simulink model "simscape_servo_model"  (R2020b)
settings: Solver=VariableStepAuto  StartTime=0.0  StopTime=10.0  RelTol=1e-3
libraries: fl_lib x7, nesl_utility x6, ee_lib x1
settings Model: Creator=akern  LastModifiedBy=akern

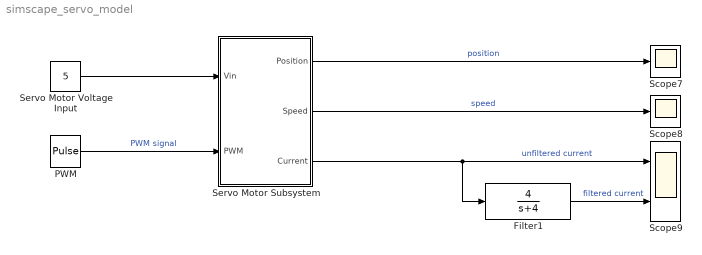
== system simscape_servo_model ==
  Filter1 : TransferFcn  Numerator=[4]  Denominator=[1 4]
  PWM : DiscretePulseGenerator  PulseType=Time based  Amplitude=5  Period=1/500  PulseWidth=50
  Scope7 : Scope
  Scope8 : Scope
  Scope9 : Scope  NumInputPorts=2
  Servo Motor Subsystem : Subsystem
  Servo Motor Voltage Input : Constant  Value=5
  wires:
  Servo Motor Subsystem/2(Speed) -> Scope8/1  "speed"
  Servo Motor Subsystem/3(Current) -> Scope9/1, Filter1/1  "unfiltered current"
  Servo Motor Voltage Input/1 -> Servo Motor Subsystem/1(Vin)
  Servo Motor Subsystem/1(Position) -> Scope7/1  "position"
  Filter1/1 -> Scope9/2  "filtered current"
  PWM/1 -> Servo Motor Subsystem/2(PWM)  "PWM signal"

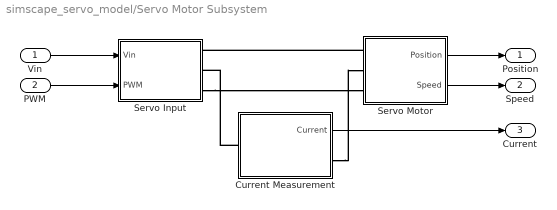
== system simscape_servo_model/Servo Motor Subsystem ==
  Vin : Inport
  PWM : Inport  Port=2
  Current Measurement : Subsystem
  Servo Input : Subsystem
  Servo Motor : Subsystem
  Position : Outport
  Speed : Outport  Port=2
  Current : Outport  Port=3
  wires:
  Servo Motor/1(Position) -> Position/1
  Vin/1 -> Servo Input/1(Vin)
  Servo Motor/2(Speed) -> Speed/1
  PWM/1 -> Servo Input/2(PWM)
  Current Measurement/1(Current) -> Current/1
  connections:
  Servo Motor/LConn1 -- Servo Input/RConn1
  Servo Input/RConn3 -- Servo Motor/LConn3
  Current Measurement/LConn1 -- Servo Input/RConn2
  Current Measurement/RConn1 -- Servo Motor/LConn2

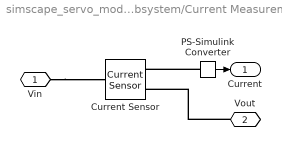
== system simscape_servo_model/Servo Motor Subsystem/Current Measurement ==
  Current Sensor : fl_lib/Electrical/Electrical Sensors/Current Sensor
  PS-Simulink Converter : nesl_utility/PS-Simulink Converter  PhysicalDomain=network_engine_domain  SubClassName=ps_output  LeftPortType=input  RightPortType=output  PseudoPeriodic=off  Frequencies=[]  Unit=inherit  AffineConversion=off
  Vin : PMIOPort  Side=Left
  Vout : PMIOPort  Port=2  Side=Right
  Current : Outport
  wires:
  PS-Simulink Converter/1 -> Current/1
  connections:
  PS-Simulink Converter/LConn1 -- Current Sensor/RConn1
  Vout/RConn1 -- Current Sensor/RConn2
  Vin/RConn1 -- Current Sensor/LConn1

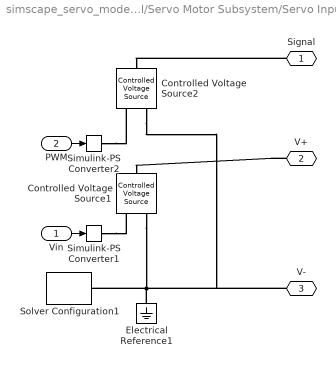
== system simscape_servo_model/Servo Motor Subsystem/Servo Input ==
  Vin : Inport
  PWM : Inport  Port=2
  Controlled Voltage Source1 : fl_lib/Electrical/Electrical Sources/Controlled Voltage Source
  Controlled Voltage Source2 : fl_lib/Electrical/Electrical Sources/Controlled Voltage Source
  Electrical Reference1 : fl_lib/Electrical/Electrical Elements/Electrical Reference
  Simulink-PS Converter1 : nesl_utility/Simulink-PS Converter  PhysicalDomain=network_engine_domain  SubClassName=ps_input  LeftPortType=input  RightPortType=output  PseudoPeriodic=off  Frequencies=[]  NoiseDistribution=none  NoiseParameters=[]  Unit=1  AffineConversion=off  FilteringAndDerivatives=provide  SimscapeFilterOrder=1  InputFilterTimeConstant=0.001  UdotUserProvided=0
  Simulink-PS Converter2 : nesl_utility/Simulink-PS Converter  PhysicalDomain=network_engine_domain  SubClassName=ps_input  LeftPortType=input  RightPortType=output  PseudoPeriodic=off  Frequencies=[]  NoiseDistribution=none  NoiseParameters=[]  Unit=1  AffineConversion=off  FilteringAndDerivatives=provide  SimscapeFilterOrder=1  InputFilterTimeConstant=0.001  UdotUserProvided=0
  Solver Configuration1 : nesl_utility/Solver Configuration  PhysicalDomain=network_engine_domain  SubClassName=solver  LeftPortType=input  RightPortType=generic  Tones=[]  Harmonics=[]  SimulateNoise=off  Profile=off  UseLocalSampling=off  EnableSwitchedLinearOptims=on  FrequencyDomain=off  UseCCode=off  RelTol=0.001  AbsTol=1e-06  MinStep=1e-09  ToWorkspace=off  RevertToSquareIcSolve=off  NumHomotopyIterations=100  PhasorMode=off  PhasorModeNumHarmonics=1  DoDC=off  ResidualTolerance=1e-09  UseLocalSolver=off  LocalSolverChoice=NE_BACKWARD_EULER_ADVANCER  LocalSolverSampleTime=0.001  DoFixedCost=off  MaxNonlinIter=3  MaxModeIter=2  ComputeImpulses=off  ImpulseIterations=2  LinearAlgebra=auto  EquationFormulation=NE_TIME_EF  DelaysMemoryBudget=1024  AutomaticFiltering=on  FilteringTimeConstant=0.001  PartitionStorageMethod=AS_NEEDED  PartitionMemoryBudget=1024  PartitionMethod=ROBUST
  Signal : PMIOPort  Side=Right
  V+ : PMIOPort  Port=2  Side=Right
  V- : PMIOPort  Port=3  Side=Right
  wires:
  PWM/1 -> Simulink-PS Converter2/1
  Vin/1 -> Simulink-PS Converter1/1
  connections:
  Controlled Voltage Source1/RConn2 -- Electrical Reference1/LConn1 -- Solver Configuration1/RConn1 -- Controlled Voltage Source2/RConn2 -- V-/RConn1
  Simulink-PS Converter1/RConn1 -- Controlled Voltage Source1/RConn1
  Signal/RConn1 -- Controlled Voltage Source2/LConn1
  Simulink-PS Converter2/RConn1 -- Controlled Voltage Source2/RConn1
  V+/RConn1 -- Controlled Voltage Source1/LConn1

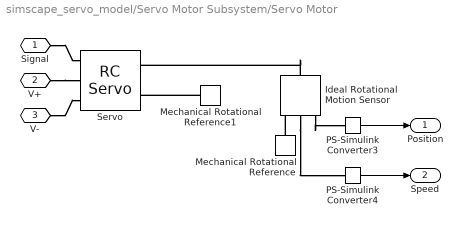
== system simscape_servo_model/Servo Motor Subsystem/Servo Motor ==
  Ideal Rotational Motion Sensor : fl_lib/Mechanical/Mechanical Sensors/Ideal Rotational Motion Sensor  wrap_angle=simscape.enum.onoff.off  offset=0 rad
  Mechanical Rotational Reference : fl_lib/Mechanical/Rotational Elements/Mechanical Rotational Reference
  Mechanical Rotational Reference1 : fl_lib/Mechanical/Rotational Elements/Mechanical Rotational Reference
  PS-Simulink Converter3 : nesl_utility/PS-Simulink Converter  PhysicalDomain=network_engine_domain  SubClassName=ps_output  LeftPortType=input  RightPortType=output  PseudoPeriodic=off  Frequencies=[]  Unit=inherit  AffineConversion=off
  PS-Simulink Converter4 : nesl_utility/PS-Simulink Converter  PhysicalDomain=network_engine_domain  SubClassName=ps_output  LeftPortType=input  RightPortType=output  PseudoPeriodic=off  Frequencies=[]  Unit=inherit  AffineConversion=off
  Servo : ee_lib/Electromechanical/Brushed Motors/RC Servo  stall_torque=2.4 kg*cm  time_60=0.28 s  nominal_voltage=4.8 V  rotational_range=[0, 180] deg  pulse_width_range=[550, 2330] us  threshold=3 V  R_s=18 kOhm  resolution=0.1 deg  angle_meas_error=0 deg  backdrive_torque=0.5 kg*cm  ratio=320  inertia=0.01 g*cm^2  endstop_angles=[-5, 185] deg  endstop_stiffness=1e6 N*m/rad  endstop_damping=0.01 N*m/(rad/s)  enable_faults=0  fault_action=1  fault_type=1  enable_temporal_fault=0  t_fault=1 s  enable_behavioral_fault=0  max_permissible_current=1 A  t_fail_on_current=1 s  angle_specify=off  angle_priority=High  angle=90 deg  angle_nominal_specify=off  angle_nominal_unit=deg  angle_nominal_value=1  w_specify=off  w_priority=High  w=0 deg/s  w_nominal_specify=off  w_nominal_unit=deg/s  w_nominal_value=1  torque_specify=off  torque_priority=None  torque=0 N*m  torque_nominal_specify=off  torque_nominal_unit=N*m  torque_nominal_value=1  pulse_width_specify=off  pulse_width_priority=Low  pulse_width=1.5 ms  i_specify=off  i_priority=None  i=0 A  i_nominal_specify=off  i_nominal_unit=A  i_nominal_value=1  i_s_specify=off  i_s_priority=None  i_s=0 A  i_s_nominal_specify=off  i_s_nominal_unit=A  i_s_nominal_value=1  motor_torque_specify=off  motor_torque_priority=None  motor_torque=0 N*m  motor_torque_nominal_specify=off  motor_torque_nominal_unit=N*m  motor_torque_nominal_value=1  power_dissipated_specify=off  power_dissipated_priority=None  power_dissipated=0 W  power_dissipated_nominal_specify=off  power_dissipated_nominal_unit=W  power_dissipated_nominal_value=1  angle_demand_specify=off  angle_demand_priority=None  angle_demand=90 deg  angle_demand_nominal_specify=off  angle_demand_nominal_unit=deg  angle_demand_nominal_value=1  faulted_specify=off  faulted_priority=None  faulted=0  faulted_nominal_specify=off  faulted_nominal_unit=1  faulted_nominal_value=1
      settings: SourceProductBaseCode=PS  InternalSimscapePortConfiguration="{\"Bottom\":[],\"Left\":[{\"id\":\"s\",\"label\":\"s\",\"type\":\"foundation.electrical.electrical\"},{\"id\":\"p\",\"label\":\"+\",\"type\":\"foundation.electrical.electrical\"},{\"id\":\"n\",\"label\":\"-\",\"type\":\"foundation.electrical.electrical\"}],\"Right\":[{\"id\":\"R\",\"label\":\"R\",\"type\":\"foundation.mechanical.rotational.rotational\"},{\"id\":\"C\",\"label\":\"C\",\"type\":\"foundation.mechanical.rotational.rotational\"}],\"Top\":[]}"
  Signal : PMIOPort  Side=Left
  V+ : PMIOPort  Port=2  Side=Left
  V- : PMIOPort  Port=3  Side=Left
  Position : Outport
  Speed : Outport  Port=2
  wires:
  PS-Simulink Converter3/1 -> Position/1
  PS-Simulink Converter4/1 -> Speed/1
  connections:
  Signal/RConn1 -- Servo/LConn1
  V-/RConn1 -- Servo/LConn3
  Ideal Rotational Motion Sensor/RConn2 -- PS-Simulink Converter4/LConn1
  Mechanical Rotational Reference/LConn1 -- Ideal Rotational Motion Sensor/RConn1
  Ideal Rotational Motion Sensor/RConn3 -- PS-Simulink Converter3/LConn1
  V+/RConn1 -- Servo/LConn2
  Ideal Rotational Motion Sensor/LConn1 -- Servo/RConn1
  Mechanical Rotational Reference1/LConn1 -- Servo/RConn2
